simulink model "controlador_hoist"  (R2023b)
settings: Solver=VariableStepAuto  StartTime=0.0  StopTime=10.0  RelTol=1e-3
undefined symbols (not defined in the file): Kd_h, Ki_h, Kp_h, Ts2
settings Model: Creator=renzo  LastModifiedBy=renzo

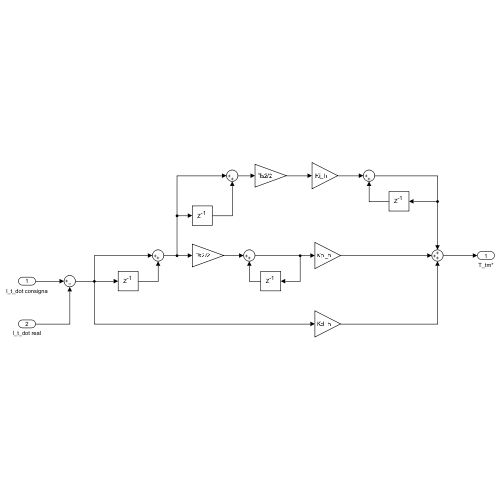
[thumbnail: Simulink's stored preview of the top-level diagram]
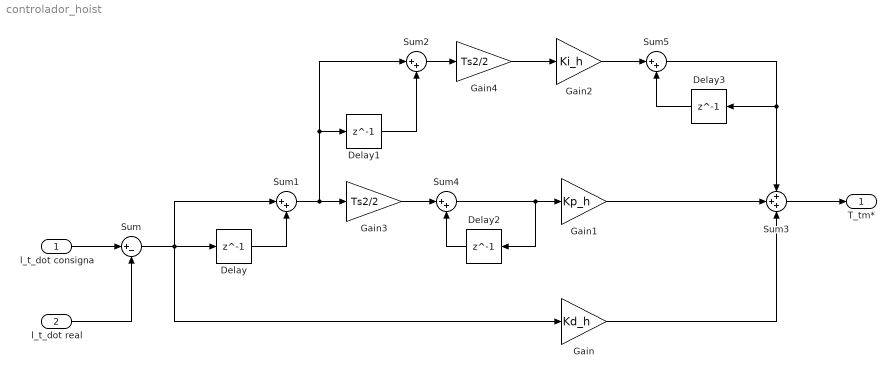
== system controlador_hoist ==
  l_t_dot consigna : Inport
  l_t_dot real : Inport  Port=2
  Delay{,1..3} (4 alike) : Delay  DelayLength=1  InitialCondition=0
  Gain : Gain  Gain=Kd_h
  Gain1 : Gain  Gain=Kp_h
  Gain2 : Gain  Gain=Ki_h
  Gain3 : Gain  Gain=Ts2/2
  Gain4 : Gain  Gain=Ts2/2
  Sum : Sum  Inputs=|+-
  Sum{1..2,4..5} (4 alike) : Sum  Inputs=|++
  Sum3 : Sum  Inputs=+++
  T_tm* : Outport
  wires:
  Sum1/1 -> Gain3/1, Sum2/1, Delay1/1
  Delay2/1 -> Sum4/2
  Delay3/1 -> Sum5/2
  Sum5/1 -> Delay3/1, Sum3/1
  Sum2/1 -> Gain4/1
  Sum3/1 -> T_tm*/1
  Delay1/1 -> Sum2/2
  Sum4/1 -> Delay2/1, Gain1/1
  Gain/1 -> Sum3/3
  Gain2/1 -> Sum5/1
  Gain4/1 -> Gain2/1
  l_t_dot real/1 -> Sum/2
  Delay/1 -> Sum1/2
  l_t_dot consigna/1 -> Sum/1
  Gain3/1 -> Sum4/1
  Sum/1 -> Sum1/1, Delay/1, Gain/1
  Gain1/1 -> Sum3/2
